simulink model "Count"  (R2022b)
settings: Solver=FixedStepAuto  StartTime=0.0  StopTime=10.0  FixedStep=0.001  RelTol=1e-3
settings Model: Creator=MAAM  LastModifiedBy=MAAM

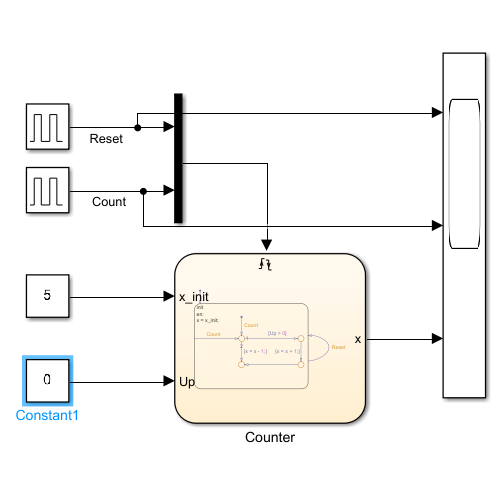
[thumbnail: Simulink's stored preview of the top-level diagram]
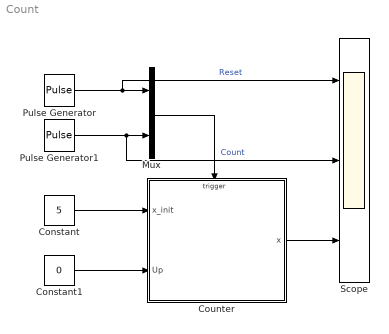
== system Count ==
  Constant : Constant  Value=5
  Constant1 : Constant  Value=0
  Counter : Stateflow chart  TreatAsAtomicUnit=on
  Mux : Mux  Inputs=2
  Pulse Generator : DiscretePulseGenerator  PulseType=Time based  Period=10  PhaseDelay=5
  Pulse Generator1 : DiscretePulseGenerator  PulseType=Time based  Period=1  PulseWidth=10
  Scope : Scope  NumInputPorts=3
  wires:
  Mux/1 -> Counter/Trigger
  Pulse Generator1/1 -> Scope/2, Mux/2  "Count"
  Pulse Generator/1 -> Scope/1, Mux/1  "Reset"
  Constant/1 -> Counter/1(x_init)
  Constant1/1 -> Counter/2(Up)
  Counter/1(x) -> Scope/3

== stateflow chart Count/Counter ==
  state init
    en:
    x = x_init;
    (default) -> (junction 16) : Count
    init -> (junction 16) [order 1] : Count
    (junction 16) -> (junction 18) [order 1] : [Up > 0]
    (junction 16) -> (junction 20) [order 2] : {x = x - 1;}
    (junction 18) -> (junction 22) : {x = x + 1;}
    (junction 22) -> (junction 20)
  (default) -> init
  init -> init [order 1] : Reset
  data: x output; x_init input; Up input
  events: Reset input FALLING_EDGE_EVENT; Count input RISING_EDGE_EVENT
